simulink model "PI_continuo2_com_wind_up_atualizado2"  (R2012b)
settings: Solver=ode45  StartTime=0.0  StopTime=100  RelTol=1e-3
settings Model: Creator=Walter  LastModifiedBy=Walter

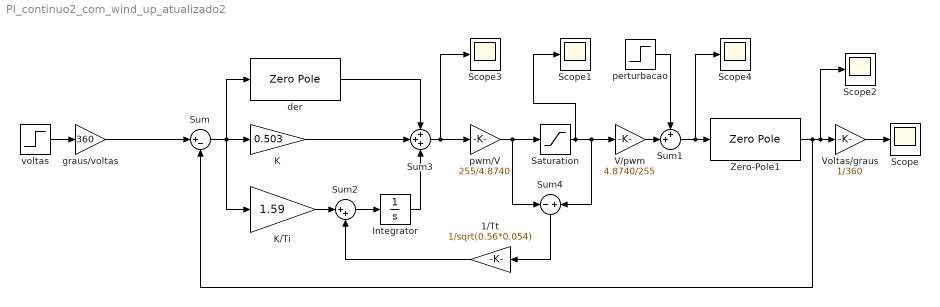
== system PI_continuo2_com_wind_up_atualizado2 ==
  1/Tt : Gain  Gain=1/sqrt(0.56*0.054)
  Integrator : Integrator
  K : Gain  Gain=0.503
  K/Ti : Gain  Gain=1.59
  Saturation : Saturate  UpperLimit=255  LowerLimit=-255
  Scope{,1..4} (5 alike) : Scope
      Scope settings: TimeRange=60  YMin=2.5  YMax=6.5
      Scope1 settings: TimeRange=100
      Scope2 settings: SaveName=ScopeData2
      Scope3 settings: TimeRange=100  SaveName=ScopeData3
      Scope4 settings: SaveName=ScopeData4
  Sum : Sum  Inputs=|+-
  Sum1 : Sum  Inputs=++|
  Sum2 : Sum  Inputs=|++
  Sum3 : Sum  Inputs=+++
  Sum4 : Sum  Inputs=-|+
  V/pwm : Gain  Gain=4.8740/255
  Voltas/graus : Gain  Gain=1/360
  Zero-Pole1 : ZeroPole  Zeros=[]  Poles=[0 -15.6250]  Gain=[1725.0719]
  der : ZeroPole  Zeros=[0]  Poles=[-200]  Gain=[0.0259/0.005]
  graus/voltas : Gain  Gain=360
  perturbacao : Step  Time=40  After=4  SampleTime=0
  pwm/V : Gain  Gain=255/4.8740
  "voltas " : Step  Time=0  After=7200/360  SampleTime=0
  wires:
  Sum/1 -> K/Ti/1, der/1, K/1
  pwm/V/1 -> Sum4/1, Saturation/1
  Saturation/1 -> Scope1/1, Sum4/2, V/pwm/1
  perturbacao/1 -> Sum1/1
  Sum1/1 -> Scope4/1, Zero-Pole1/1
  "voltas "/1 -> graus/voltas/1
  Zero-Pole1/1 -> Sum/2, Scope2/1, Voltas/graus/1
  graus/voltas/1 -> Sum/1
  Voltas/graus/1 -> Scope/1
  Sum3/1 -> Scope3/1, pwm/V/1
  V/pwm/1 -> Sum1/2
  K/Ti/1 -> Sum2/1
  Sum2/1 -> Integrator/1
  K/1 -> Sum3/2
  der/1 -> Sum3/1
  Integrator/1 -> Sum3/3
  1/Tt/1 -> Sum2/2
  Sum4/1 -> 1/Tt/1
